simulink model "tarmodel"  (R2023a)
settings: Solver=ode3  StartTime=0.0  StopTime=10.0  RelTol=1e-3
Description:
  | ###CmwHarnessModel###
settings Model: Creator=chin.j  LastModifiedBy=user6.gaio
settings SolverCC: AlgebraicLoopSolver=TrustRegion
settings DataIOCC: SaveOutput=off  SaveTime=off  ReturnWorkspaceOutputs=off
settings OptimizationCC: LifeSpan=inf
settings DebuggingCC: UnconnectedInputMsg=warning  UnconnectedOutputMsg=warning  UnconnectedLineMsg=warning  StrictBusMsg=ErrorOnBusTreatedAsVector  SFExecutionAtInitializationDiag=none  ArithmeticOperatorsInVariantConditions=warning
settings HardwareCC: ProdBitPerSizeT=32  ProdBitPerPtrDiffT=32  ProdWordSize=32  ProdHWDeviceType=Specified
settings SFSimCC: CustomCodeUndefinedFunction=UseInterfaceOnly
settings CodeAppCC: StateflowObjectComments=on

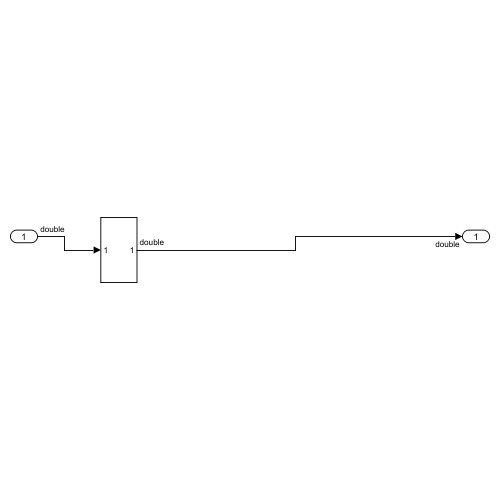
[thumbnail: Simulink's stored preview of the top-level diagram]
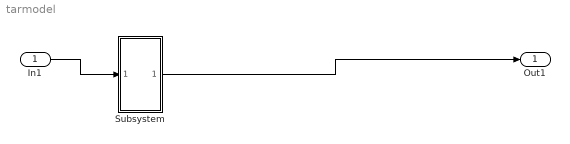
== system tarmodel ==
  In1 : Inport  OutDataTypeStr=double  PortDimensions=1  Interpolate=off
  Subsystem : Subsystem
  Out1 : Outport  OutDataTypeStr=double
  wires:
  In1/1 -> Subsystem/1(In1)
  Subsystem/1(Out1) -> Out1/1

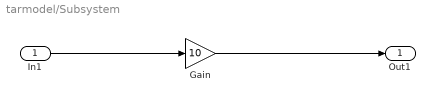
== system tarmodel/Subsystem ==
  In1 : Inport
  Gain : Gain  Gain=10
  Out1 : Outport
  wires:
  In1/1 -> Gain/1
  Gain/1 -> Out1/1
